simulink model "my_model"  (R2023a)
settings: Solver=VariableStepAuto  StartTime=0.0  StopTime=10.0  RelTol=1e-3
settings Model: Creator=fy153  LastModifiedBy=fy153

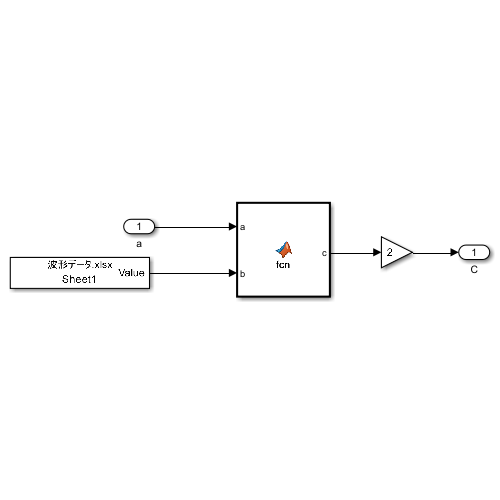
[thumbnail: Simulink's stored preview of the top-level diagram]
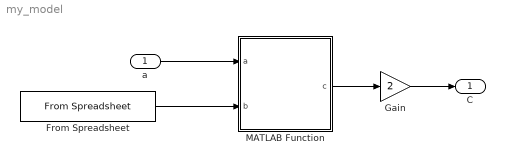
== system my_model ==
  a : Inport
  From Spreadsheet : FromSpreadsheet  FileName=波形データ.xlsx
  Gain : Gain  Gain=2
  MATLAB Function : MATLAB Function  TreatAsAtomicUnit=on
  C : Outport
  wires:
  a/1 -> MATLAB Function/1(a)
  From Spreadsheet/1 -> MATLAB Function/2(b)
  MATLAB Function/1(c) -> Gain/1
  Gain/1 -> C/1

== matlab function my_model/MATLAB Function ==
  data: a input; c output; b input
function c = fcn(a, b)

c = my_func(a, b);

end
